simulink model "c2_6_1zhuangtaiguancefankuikongzhiqi"  (R2019b)
settings: Solver=VariableStepAuto  StartTime=0.0  StopTime=30  RelTol=1e-3
settings Model: Creator=wy151  LastModifiedBy=wy151

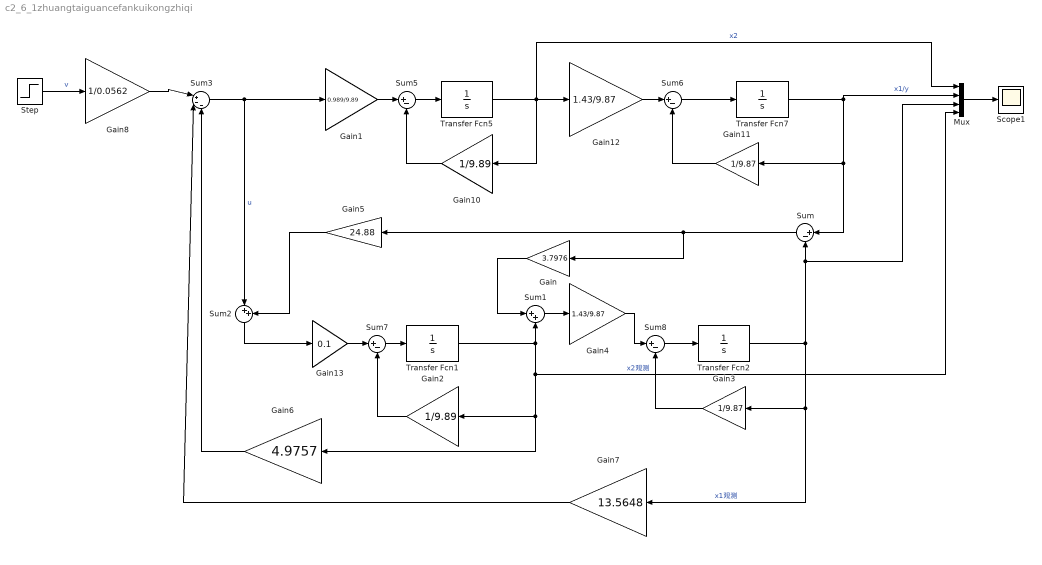
== system c2_6_1zhuangtaiguancefankuikongzhiqi ==
  Gain : Gain  Gain=3.7976
  Gain1 : Gain  Gain=0.989/9.89
  Gain10 : Gain  Gain=1/9.89
  Gain11 : Gain  Gain=1/9.87
  Gain12 : Gain  Gain=1.43/9.87
  Gain13 : Gain  Gain=0.1
  Gain2 : Gain  Gain=1/9.89
  Gain3 : Gain  Gain=1/9.87
  Gain4 : Gain  Gain=1.43/9.87
  Gain5 : Gain  Gain=24.88
  Gain6 : Gain  Gain=4.9757
  Gain7 : Gain  Gain=13.5648
  Gain8 : Gain  Gain=1/0.0562
  Mux : Mux
  Scope1 : Scope
  Step : Step  SampleTime=0
  Sum{,5..8} (5 alike) : Sum  Inputs=|+-
  Sum1 : Sum  Inputs=|++
  Sum2 : Sum  Inputs=|++
  Sum3 : Sum  Inputs=|+--
  Transfer Fcn{1..2,5,7} (4 alike) : TransferFcn  Denominator=[1 0]
  wires:
  Gain4/1 -> Sum8/1
  Gain12/1 -> Sum6/1
  Sum8/1 -> Transfer Fcn2/1
  Gain2/1 -> Sum7/2
  Sum2/1 -> Gain13/1
  Sum1/1 -> Gain4/1
  Gain3/1 -> Sum8/2
  Gain1/1 -> Sum5/1
  Sum7/1 -> Transfer Fcn1/1
  Gain11/1 -> Sum6/2
  Sum6/1 -> Transfer Fcn7/1
  Gain/1 -> Sum1/1
  Gain13/1 -> Sum7/1
  Gain10/1 -> Sum5/2
  Transfer Fcn5/1 -> Mux/1, Gain12/1, Gain10/1  "x2"
  Gain5/1 -> Sum2/2
  Sum/1 -> Gain5/1, Gain/1
  Transfer Fcn7/1 -> Sum/1, Gain11/1, Mux/2  "x1/y"
  Sum5/1 -> Transfer Fcn5/1
  Transfer Fcn2/1 -> Sum/2, Mux/3, Gain7/1, Gain3/1  "x1观测"
  Transfer Fcn1/1 -> Gain6/1, Gain2/1, Mux/4, Sum1/2  "x2观测"
  Sum3/1 -> Sum2/1, Gain1/1  "u"
  Gain6/1 -> Sum3/3
  Gain7/1 -> Sum3/2
  Gain8/1 -> Sum3/1
  Step/1 -> Gain8/1  "v"
  Mux/1 -> Scope1/1
